simulink model "problem1"  (R2020a)
settings: Solver=VariableStepAuto  StartTime=0.0  StopTime=10.0  RelTol=1e-3
settings Model: Creator=HP  LastModifiedBy=HP

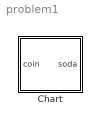
== system problem1 ==
  Chart : Stateflow chart  TreatAsAtomicUnit=on

== stateflow chart problem1/Chart ==
  state Got_0
  state Got_Nickel
  state Got_Dime
  Got_0 -> Got_Nickel [order 1] : [coin==1]{soda=0}
  (default) -> Got_0
  Got_Dime -> Got_0 [order 1] : [coin==1]{soda=1}
  Got_0 -> Got_Dime [order 2] : [coin==2]{soda=0}
  Got_Nickel -> Got_0 [order 2] : [coin==2]{soda=1}
  Got_Nickel -> Got_Dime [order 1] : [coin==1]{soda=0}
  Got_Dime -> Got_Nickel [order 2] : [coin==2]{soda=1}
  data: coin input; soda output
